simulink model "mysdof"  (Simulink 9.2)
settings: Solver=ode3  StartTime=0.0  StopTime=10.0  FixedStep=0.002  RelTol=1e-3
settings Model: Creator=Billy  LastModifiedBy=Billy
settings DataIOCC: LimitDataPoints=off  SaveFormat=Dataset  SignalLoggingSaveFormat=Dataset
settings OptimizationCC: LifeSpan=auto
settings DebuggingCC: UnderspecifiedInitializationDetection=Simplified  MergeDetectMultiDrivingBlocksExec=error  FcnCallInpInsideContextMsg=error  StateNameClashWarn=none  SFUnexpectedBacktrackingDiag=error  SFNoUnconditionalDefaultTransitionDiag=error  SFExecutionAtInitializationDiag=warning
settings HardwareCC: ProdBitPerPointer=64  ProdBitPerSizeT=64  ProdBitPerPtrDiffT=64  ProdLargestAtomicFloat=Float  ProdIntDivRoundTo=Zero  ProdEndianess=LittleEndian  ProdWordSize=64  ProdHWDeviceType=Intel->x86-64 (Windows64)
settings ModelReferenceCC: PropagateSignalLabelsOutOfModel=on
settings SFSimCC: SimUseLocalCustomCode=on
settings RTWCC: RTWUseLocalCustomCode=on
settings CodeAppCC: StateflowObjectComments=off
settings GRTTargetCC: TargetLangStandard=C99 (ISO)  GeneratePreprocessorConditionals=Use local settings  CombineOutputUpdateFcns=on  GRTInterface=off
settings ConfigComp: CovMetricSettings=dwe  CovHtmlReporting=off  CovSaveCumulativeToWorkspaceVar=off  CovSaveSingleToWorkspaceVar=off  CovExternalEMLEnable=on

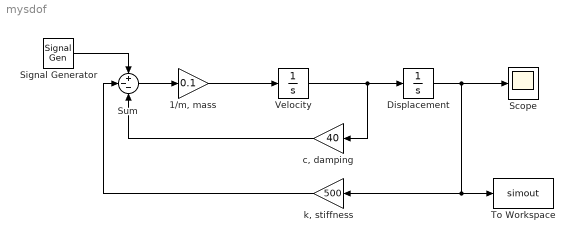
== system mysdof ==
  "1/m, mass" : Gain  Gain=0.1
  Displacement : Integrator  InitialCondition=0.01
  Scope : Scope
  Signal Generator : SignalGenerator  WaveForm=square  Amplitude=0  Frequency=0.2
  Sum : Sum  Inputs=+--
  To Workspace : ToWorkspace  VariableName=simout  SampleTime=-1
  Velocity : Integrator  InitialCondition=1
  "c, damping" : Gain  Gain=40
  "k, stiffness " : Gain  Gain=500
  wires:
  Velocity/1 -> "c, damping"/1, Displacement/1
  "1/m, mass"/1 -> Velocity/1
  Displacement/1 -> Scope/1, To Workspace/1, "k, stiffness "/1
  Sum/1 -> "1/m, mass"/1
  Signal Generator/1 -> Sum/1
  "c, damping"/1 -> Sum/3
  "k, stiffness "/1 -> Sum/2
